simulink model "P413_2_model"  (R2021a)
settings: Solver=VariableStepAuto  StartTime=0.0  StopTime=tspan(end)  RelTol=1e-3
values from neighbouring files (symbols this model uses):
  AR = params(1).Value    [P413_2_clima.m]
  beta = 0    [P413_2_clima.m]
  gamma = 0    [P413_2_clima.m]
libraries: HORTISIM x4
settings Model: OrderedModelArguments=off  Creator=djoroya  LastModifiedBy=djoroya
settings DataIOCC: ExternalInput=tp3276776d_8610_4451_82d6_0aeb35eee2de(1)  LoadExternalInput=on  OutputOption=AdditionalOutputTimes  OutputTimes=SDO_OutputTimes  ReturnWorkspaceOutputsName=SDOSimTest_Log

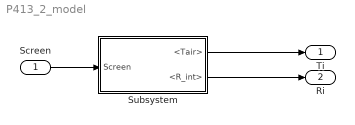
== system P413_2_model ==
  Screen : Inport
  Subsystem : Subsystem
  Ti : Outport
  Ri : Outport  Port=2
  wires:
  Subsystem/1(<Tair>) -> Ti/1
  Subsystem/2(<R_int>) -> Ri/1
  Screen/1 -> Subsystem/1(Screen)

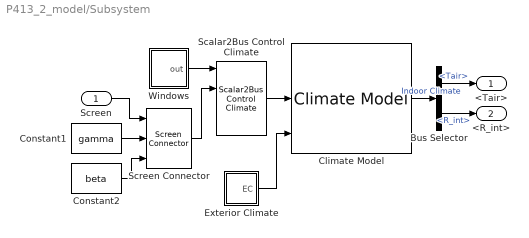
== system P413_2_model/Subsystem ==
  Screen : Inport
  Bus Selector : BusSelector  OutputSignals=Temp.Tair,QS.R_int
  Climate Model : HORTISIM/Climate/Models/Climate Model  hour0=x0_ic.hour0  G0=x0_ic.G0  T0=x0_ic.T0  H=p_ic.H  A_f=p_ic.A_f  A_c=p_ic.A_c  minWindows=p_ic.minWindows  lam_s=p_ic.lam_s  c_s=p_ic.c_s  l_s=p_ic.l_s  rhod_s=p_ic.rhod_s  int_air_speed=p_ic.int_air_speed  alpha_i=p_ic.alpha_i  alpha_c=p_ic.alpha_c  tau_c=p_ic.tau_c  alpha_f=p_ic.alpha_f  d_c=p_ic.d_c  cd_c=p_ic.cd_c  T_ss=p_ic.T_ss
      settings: SourceProductName=Horti Simulator
  Constant1 : Constant  Value=gamma
  Constant2 : Constant  Value=beta
  Exterior Climate : Subsystem
  Scalar2Bus Control Climate : HORTISIM/Other  Functions/Scalar2Bus  Control Climate  SystemSampleTime=-1  VariantActivationTime=update diagram  Latency=0  AutoFrameSizeCalculation=off
      settings: SourceProductName=Horti Simulator
  Screen Connector : HORTISIM/Other  Functions/Screen Connector  SystemSampleTime=-1  VariantActivationTime=update diagram  Latency=0  AutoFrameSizeCalculation=off
      settings: SourceProductName=Horti Simulator
  Windows : Subsystem
  <Tair> : Outport
  <R_int> : Outport  Port=2
  wires:
  Bus Selector/2 -> <R_int>/1  "<R_int>"
  Screen Connector/1 -> Scalar2Bus Control Climate/2
  Bus Selector/1 -> <Tair>/1  "<Tair>"
  Climate Model/1 -> Bus Selector/1  "Indoor Climate"
  Scalar2Bus Control Climate/1 -> Climate Model/2
  Exterior Climate/1(EC) -> Climate Model/3
  Screen/1 -> Screen Connector/1
  Constant1/1 -> Screen Connector/2
  Constant2/1 -> Screen Connector/3
  Windows/1(out) -> Scalar2Bus Control Climate/1

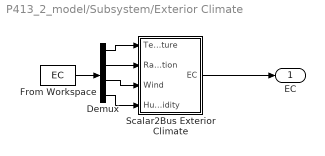
== system P413_2_model/Subsystem/Exterior Climate ==
  Demux : Demux
  From Workspace : FromWorkspace  VariableName=EC
  Scalar2Bus Exterior Climate : Subsystem
  EC : Outport
  wires:
  Demux/3 -> Scalar2Bus Exterior Climate/3(Wind)
  Demux/2 -> Scalar2Bus Exterior Climate/2(Radiation)
  Scalar2Bus Exterior Climate/1(EC) -> EC/1
  Demux/1 -> Scalar2Bus Exterior Climate/1(Temperature)
  Demux/4 -> Scalar2Bus Exterior Climate/4(Humidity)
  From Workspace/1 -> Demux/1

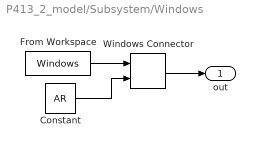
== system P413_2_model/Subsystem/Windows ==
  Constant : Constant  Value=AR
  From Workspace : FromWorkspace  VariableName=Windows
  Windows Connector : HORTISIM/Other  Functions/Windows Connector  SystemSampleTime=-1  VariantActivationTime=update diagram  Latency=0  AutoFrameSizeCalculation=off
      settings: SourceProductName=Horti Simulator
  out : Outport
  wires:
  Windows Connector/1 -> out/1
  From Workspace/1 -> Windows Connector/1
  Constant/1 -> Windows Connector/2

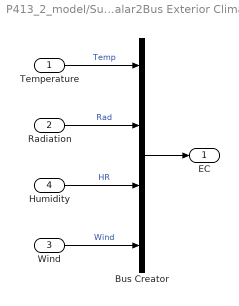
== system P413_2_model/Subsystem/Exterior Climate/Scalar2Bus Exterior Climate ==
  Temperature : Inport
  Radiation : Inport  Port=2
  Wind : Inport  Port=3
  Humidity : Inport  Port=4
  Bus Creator : BusCreator  Inputs=4
  EC : Outport
  wires:
  Humidity/1 -> Bus Creator/3  "HR"
  Wind/1 -> Bus Creator/4  "Wind"
  Temperature/1 -> Bus Creator/1  "Temp"
  Bus Creator/1 -> EC/1
  Radiation/1 -> Bus Creator/2  "Rad"
